simulink model "L2_lorenz"  (R2023b)
settings: Solver=FixedStepAuto  StartTime=0.0  StopTime=30  FixedStep=0.001  RelTol=1e-3
settings Model: Creator=Basia  LastModifiedBy=Joanna

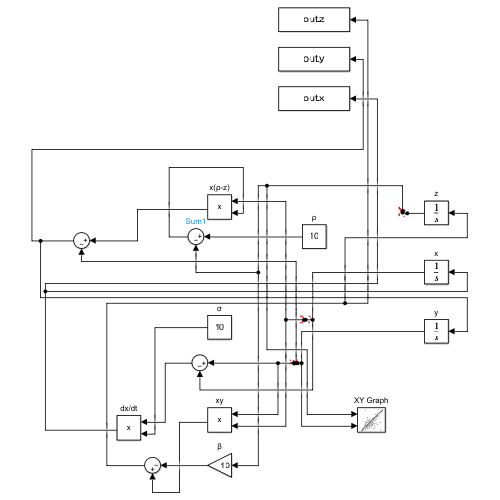
[thumbnail: Simulink's stored preview of the top-level diagram]
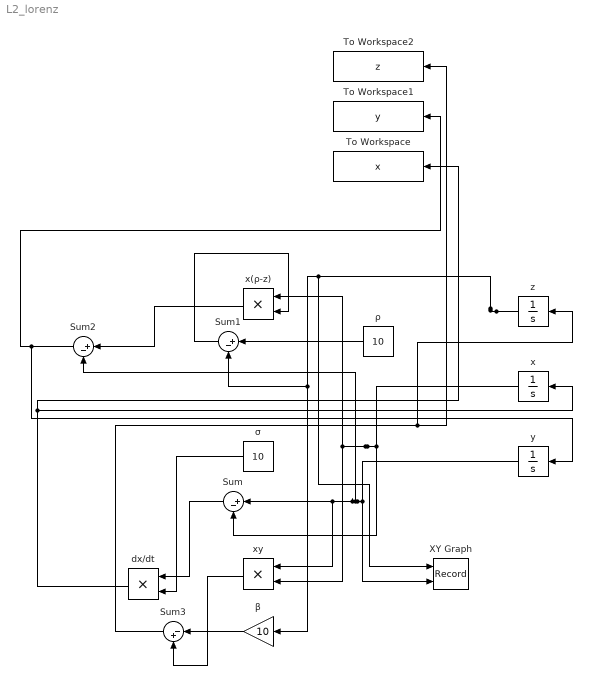
== system L2_lorenz ==
  Sum : Sum  Inputs=|+-
  Sum1 : Sum  Inputs=|+-
  Sum2 : Sum  Inputs=|+-
  Sum3 : Sum  Inputs=|-+
  To Workspace : ToWorkspace  VariableName=x  SampleTime=-1
  To Workspace1 : ToWorkspace  VariableName=y  SampleTime=-1
  To Workspace2 : ToWorkspace  VariableName=z  SampleTime=-1
  XY Graph : Record  FileSettingsInternal="{\"entries\":[{\"content\":{\"excelSettings\":{\"content\":{},\"type\":\"Streamout.ExcelSettings\"}},\"type\":\"Streamout.FileSettingStorage\",\"uuid\":\"\"}],\"packageUris\":[\"http:\\/\\/schema.mathworks.com\\/mf0\\/streamout_blocks\\/R2020a\"],\"version\":\"1.0\"}"  Layout=[1 1]  SignalsInternal="{\"entries\":[{\"content\":{\"signals\":[{\"content\":{\"blockPath\":[],\"dimensions\":[1],\"domain\":\"\",\"lineColor\":\"#a2142f\",\"plots\":[ 1 ],\"port\":1,\"sid\":[\"\"],\"signalID\":1,\"signalName\":\"z\"},\"type\":\"RecordBlkView.Signal\",\"uuid\":\"\"},{\"content\":{\"blockPath\":[],\"dimensions\":[1],\"domain\":\"\",\"lineColor\":\"#139fff\",\"plots\":[ 1 ],\"port\":2,\"sid\":[\"\"],\"signalID\":2,\"signalName\":\"y\"},\"type\":\"RecordBlkView.Signal\",\"uuid\":\"\"}]},\"type\":\"RecordBlkView.InputSignals\",\"uuid\":\"\"}],\"packageUris\":[\"http:\\/\\/schema.mathworks.com\\/mf0\\/streamout_blocks\\/R2020a\"],\"version\":\"1.0\"}"  CompatibilityTag=XY
  dx/dt : Product
  x : Integrator  InitialCondition=1
  x(ρ-z) : Product
  xy : Product
  y : Integrator  InitialCondition=1
  z : Integrator  InitialCondition=1
  β : Gain  Gain=10
  ρ : Constant  Value=10
  σ : Constant  Value=10
  wires:
  y/1 -> Sum/1, xy/1, Sum2/2, XY Graph/2
  x/1 -> x(ρ-z)/1, xy/2, Sum/2
  Sum/1 -> dx/dt/1
  σ/1 -> dx/dt/2
  ρ/1 -> Sum1/1
  z/1 -> β/1, Sum1/2, XY Graph/1
  Sum1/1 -> x(ρ-z)/2
  x(ρ-z)/1 -> Sum2/1
  dx/dt/1 -> To Workspace/1, x/1
  Sum2/1 -> To Workspace1/1, y/1
  β/1 -> Sum3/1
  xy/1 -> Sum3/2
  Sum3/1 -> z/1, To Workspace2/1
